simulink model "square_wave_gen_higher_res"  (R2018b)
settings: Solver=VariableStepAuto  StartTime=0.0  StopTime=5e-3  RelTol=1e-3
settings Model: Creator=sangh  LastModifiedBy=sangh

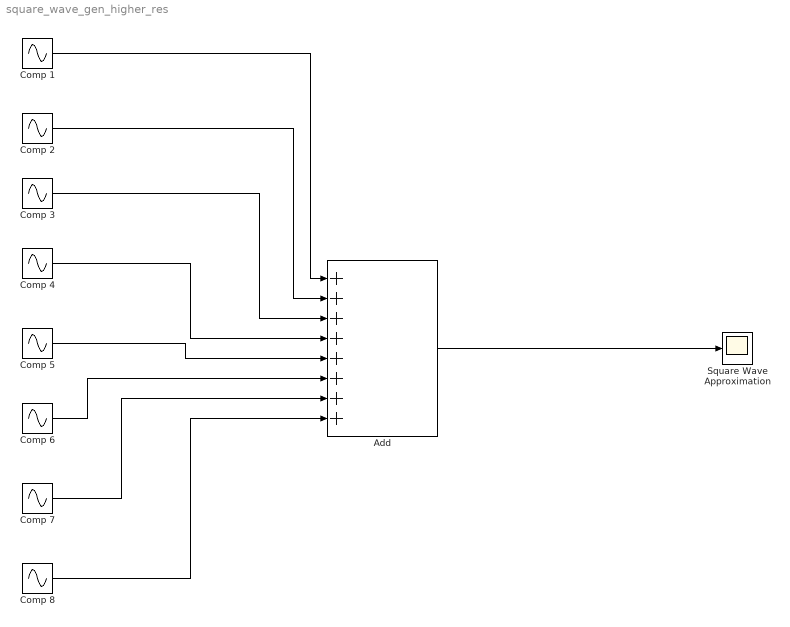
== system square_wave_gen_higher_res ==
  Add : Sum  Inputs=++++++++
  Comp 1 : Sin  Amplitude=4/pi  Frequency=2*pi*500  SampleTime=0.25e-6
  Comp 2 : Sin  Amplitude=4/(3*pi)  Frequency=2*pi*1500  SampleTime=0.25e-6
  Comp 3 : Sin  Amplitude=4/(5*pi)  Frequency=2*pi*2500  SampleTime=0.25e-6
  Comp 4 : Sin  Amplitude=4/(7*pi)  Frequency=2*pi*3500  SampleTime=0.25e-6
  Comp 5 : Sin  Amplitude=4/(9*pi)  Frequency=2*pi*4500  SampleTime=0.25e-6
  Comp 6 : Sin  Amplitude=4/(11*pi)  Frequency=2*pi*5500  SampleTime=0.25e-6
  Comp 7 : Sin  Amplitude=4/(13*pi)  Frequency=2*pi*6500  SampleTime=0.25e-6
  Comp 8 : Sin  Amplitude=4/(15*pi)  Frequency=2*pi*7500  SampleTime=0.25e-6
  Square Wave Approximation : Scope
  wires:
  Comp 8/1 -> Add/8
  Comp 7/1 -> Add/7
  Comp 6/1 -> Add/6
  Comp 5/1 -> Add/5
  Comp 4/1 -> Add/4
  Comp 3/1 -> Add/3
  Comp 2/1 -> Add/2
  Comp 1/1 -> Add/1
  Add/1 -> Square Wave Approximation/1
